simulink model "Adap_ob_CIDA_3_ODR_CFC"  (R2021b)
settings: Solver=ode5  StartTime=0.0  StopTime=90.0  FixedStep=0.02  RelTol=1e-3
settings Model: Creator=a1752760  LastModifiedBy=a1752760

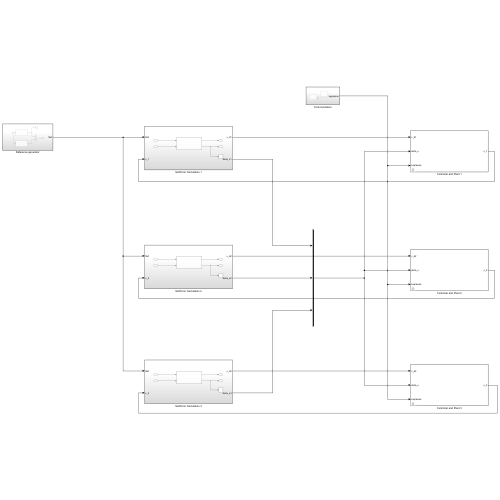
[thumbnail: Simulink's stored preview of the top-level diagram]
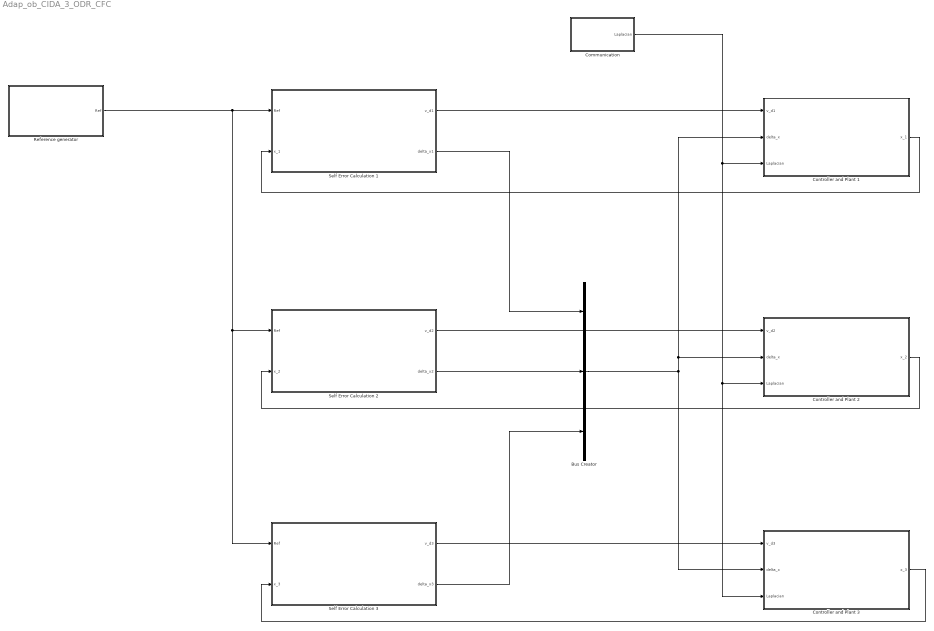
== system Adap_ob_CIDA_3_ODR_CFC ==
  Bus Creator : BusCreator  Inputs=3
  Communication : Subsystem
  Controller and Plant 1 : Subsystem  mask{InitialCondition=[-0.6;0.3;-pi/4], UpperLimit=0.2, LowerLimit=-0.2}
      mask prompts: InitialCondition "Simulink:blkprm_prompts:IntegratorInitCond"; UpperLimit "Simulink:blkprm_prompts:SaturateUpLim"; LowerLimit "Simulink:blkprm_prompts:SaturateLowLim"
      mask TypeOptions InitialCondition: x_int/InitialCondition
      mask TypeOptions UpperLimit: Saturation/UpperLimit
      mask TypeOptions LowerLimit: Saturation/LowerLimit
      mask DialogControl InitialCondition Prompt: Initial condition:
      mask DialogControl UpperLimit Prompt: Upper limit:
      mask DialogControl LowerLimit Prompt: Lower limit:
  Controller and Plant 2 : Subsystem  mask{InitialCondition=[0.1;1.4;pi/5], UpperLimit=0.2, LowerLimit=-0.2}
      mask prompts: InitialCondition "Simulink:blkprm_prompts:IntegratorInitCond"; UpperLimit "Simulink:blkprm_prompts:SaturateUpLim"; LowerLimit "Simulink:blkprm_prompts:SaturateLowLim"
      mask TypeOptions InitialCondition: x_int/InitialCondition
      mask TypeOptions UpperLimit: Saturation/UpperLimit
      mask TypeOptions LowerLimit: Saturation/LowerLimit
      mask DialogControl InitialCondition Prompt: Initial condition:
      mask DialogControl UpperLimit Prompt: Upper limit:
      mask DialogControl LowerLimit Prompt: Lower limit:
  Controller and Plant 3 : Subsystem  mask{InitialCondition=[1.1;0;pi/10], UpperLimit=0.2, LowerLimit=-0.2}
      mask prompts: InitialCondition "Simulink:blkprm_prompts:IntegratorInitCond"; UpperLimit "Simulink:blkprm_prompts:SaturateUpLim"; LowerLimit "Simulink:blkprm_prompts:SaturateLowLim"
      mask TypeOptions InitialCondition: x_int/InitialCondition
      mask TypeOptions UpperLimit: Saturation/UpperLimit
      mask TypeOptions LowerLimit: Saturation/LowerLimit
      mask DialogControl InitialCondition Prompt: Initial condition:
      mask DialogControl UpperLimit Prompt: Upper limit:
      mask DialogControl LowerLimit Prompt: Lower limit:
  Reference generator : Subsystem
  Self Error Calculation 1 : Subsystem
  Self Error Calculation 2 : Subsystem
  Self Error Calculation 3 : Subsystem
  wires:
  Communication/1(Laplacian) -> Controller and Plant 3/3(Laplacian), Controller and Plant 2/3(Laplacian), Controller and Plant 1/3(Laplacian)
  Self Error Calculation 1/2(delta_x1) -> Bus Creator/1
  Bus Creator/1 -> Controller and Plant 3/2(delta_x), Controller and Plant 2/2(delta_x), Controller and Plant 1/2(delta_x)
  Self Error Calculation 2/1(v_d2) -> Controller and Plant 2/1(v_d2)
  Self Error Calculation 2/2(delta_x2) -> Bus Creator/2
  Self Error Calculation 3/2(delta_x3) -> Bus Creator/3
  Self Error Calculation 3/1(v_d3) -> Controller and Plant 3/1(v_d3)
  Controller and Plant 2/1(x_2) -> Self Error Calculation 2/2(x_2)
  Controller and Plant 3/1(x_3) -> Self Error Calculation 3/2(x_3)
  Reference generator/1(Ref) -> Self Error Calculation 3/1(Ref), Self Error Calculation 2/1(Ref), Self Error Calculation 1/1(Ref)
  Controller and Plant 1/1(x_1) -> Self Error Calculation 1/2(x_1)
  Self Error Calculation 1/1(v_d1) -> Controller and Plant 1/1(v_d1)

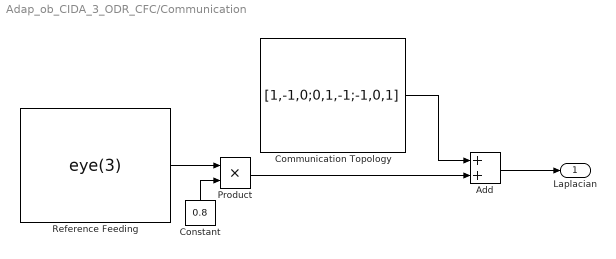
== system Adap_ob_CIDA_3_ODR_CFC/Communication ==
  Add : Sum
  Communication Topology : Constant  Value=[1,-1,0;0,1,-1;-1,0,1]  VectorParams1D=off
  Constant : Constant  Value=0.8  VectorParams1D=off
  Product : Product
  Reference Feeding : Constant  Value=eye(3)  VectorParams1D=off
  Laplacian : Outport  VectorParamsAs1DForOutWhenUnconnected=off
  wires:
  Constant/1 -> Product/2
  Reference Feeding/1 -> Product/1
  Communication Topology/1 -> Add/1
  Product/1 -> Add/2
  Add/1 -> Laplacian/1

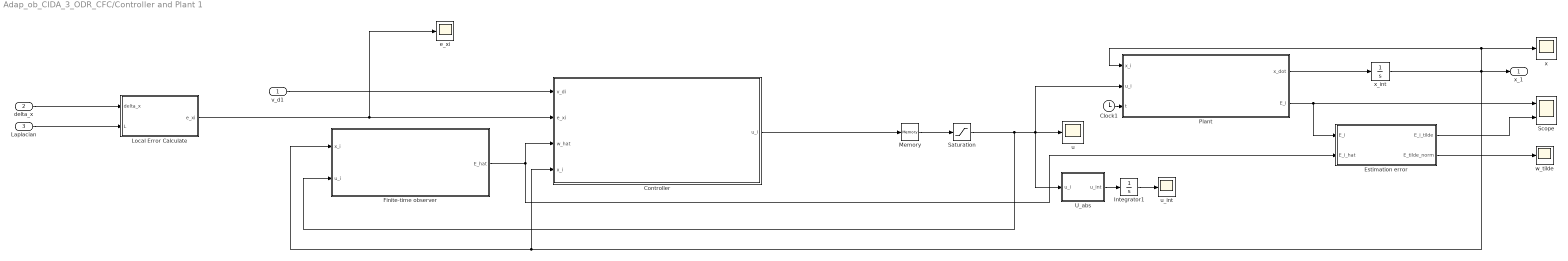
== system Adap_ob_CIDA_3_ODR_CFC/Controller and Plant 1 ==
  v_d1 : Inport
  delta_x : Inport  Port=2
  Laplacian : Inport  Port=3
  Clock1 : Clock
  Controller : Subsystem
  Estimation error : MATLAB Function  TreatAsAtomicUnit=on
  Finite-time observer : Subsystem  mask{InitialCondition=[-0.6;0.3;-pi/4]}
      mask prompts: InitialCondition "Simulink:blkprm_prompts:IntegratorInitCond"
      mask TypeOptions InitialCondition: Integrator/InitialCondition
      mask DialogControl InitialCondition Prompt: Initial condition:
  Integrator1 : Integrator
  Local Error Calculate : MATLAB Function  TreatAsAtomicUnit=on
  Memory : Memory  InitialCondition=[0;0;0]
  Plant : MATLAB Function  TreatAsAtomicUnit=on
  Saturation : Saturate  UpperLimit=UpperLimit  LowerLimit=LowerLimit
  Scope : Scope  NumInputPorts=2
  U_abs : MATLAB Function  TreatAsAtomicUnit=on
  e_xi : Scope
  u : Scope
  u_int : Scope
  w_tilde : Scope
  x : Scope
  x_int : Integrator  InitialCondition=InitialCondition
  x_1 : Outport
  wires:
  Plant/2(E_i) -> Scope/1, Estimation error/1(E_i)
  Finite-time observer/1(E_hat) -> Estimation error/2(E_i_hat), Controller/3(w_hat)
  Clock1/1 -> Plant/3(t)
  Plant/1(x_dot) -> x_int/1
  Memory/1 -> Saturation/1
  x_int/1 -> x_1/1, Plant/1(x_i), x/1, Finite-time observer/1(x_i), Controller/4(x_i)
  v_d1/1 -> Controller/1(v_di)
  Controller/1(u_i) -> Memory/1
  Local Error Calculate/1(e_xi) -> Controller/2(e_xi), e_xi/1
  delta_x/1 -> Local Error Calculate/1(delta_x)
  Laplacian/1 -> Local Error Calculate/2(L)
  Saturation/1 -> Finite-time observer/2(u_i), U_abs/1(u_i), Plant/2(u_i), u/1
  Integrator1/1 -> u_int/1
  U_abs/1(u_int) -> Integrator1/1
  Estimation error/2(E_tilde_norm) -> w_tilde/1
  Estimation error/1(E_i_tilde) -> Scope/2

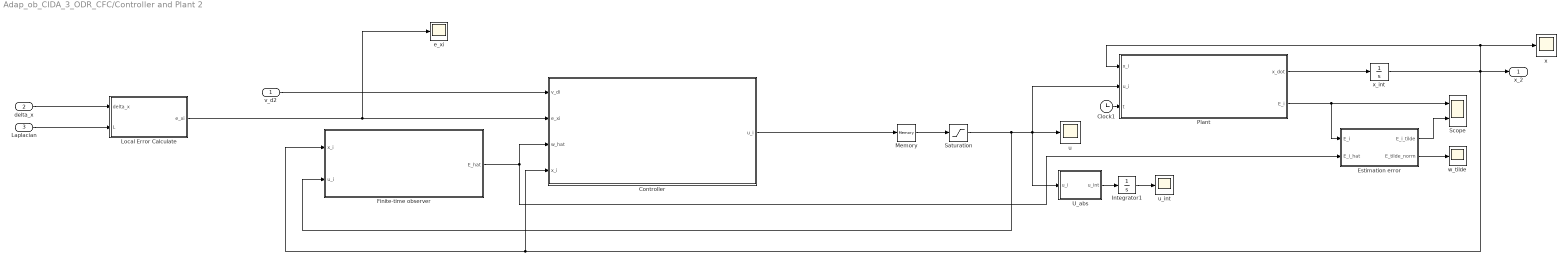
== system Adap_ob_CIDA_3_ODR_CFC/Controller and Plant 2 ==
  v_d2 : Inport
  delta_x : Inport  Port=2
  Laplacian : Inport  Port=3
  Clock1 : Clock
  Controller : Subsystem
  Estimation error : MATLAB Function  TreatAsAtomicUnit=on
  Finite-time observer : Subsystem  mask{InitialCondition=[0.1;1.4;pi/5]}
      mask prompts: InitialCondition "Simulink:blkprm_prompts:IntegratorInitCond"
      mask TypeOptions InitialCondition: Integrator/InitialCondition
      mask DialogControl InitialCondition Prompt: Initial condition:
  Integrator1 : Integrator
  Local Error Calculate : MATLAB Function  TreatAsAtomicUnit=on
  Memory : Memory  InitialCondition=[0;0;0]
  Plant : MATLAB Function  TreatAsAtomicUnit=on
  Saturation : Saturate  UpperLimit=UpperLimit  LowerLimit=LowerLimit
  Scope : Scope  NumInputPorts=2
  U_abs : MATLAB Function  TreatAsAtomicUnit=on
  e_xi : Scope
  u : Scope
  u_int : Scope
  w_tilde : Scope
  x : Scope
  x_int : Integrator  InitialCondition=InitialCondition
  x_2 : Outport
  wires:
  Plant/2(E_i) -> Estimation error/1(E_i), Scope/1
  Finite-time observer/1(E_hat) -> Controller/3(w_hat), Estimation error/2(E_i_hat)
  Clock1/1 -> Plant/3(t)
  Plant/1(x_dot) -> x_int/1
  Memory/1 -> Saturation/1
  x_int/1 -> x_2/1, Plant/1(x_i), x/1, Controller/4(x_i), Finite-time observer/1(x_i)
  v_d2/1 -> Controller/1(v_di)
  Controller/1(u_i) -> Memory/1
  Local Error Calculate/1(e_xi) -> Controller/2(e_xi), e_xi/1
  delta_x/1 -> Local Error Calculate/1(delta_x)
  Laplacian/1 -> Local Error Calculate/2(L)
  Integrator1/1 -> u_int/1
  Saturation/1 -> Finite-time observer/2(u_i), U_abs/1(u_i), Plant/2(u_i), u/1
  U_abs/1(u_int) -> Integrator1/1
  Estimation error/2(E_tilde_norm) -> w_tilde/1
  Estimation error/1(E_i_tilde) -> Scope/2

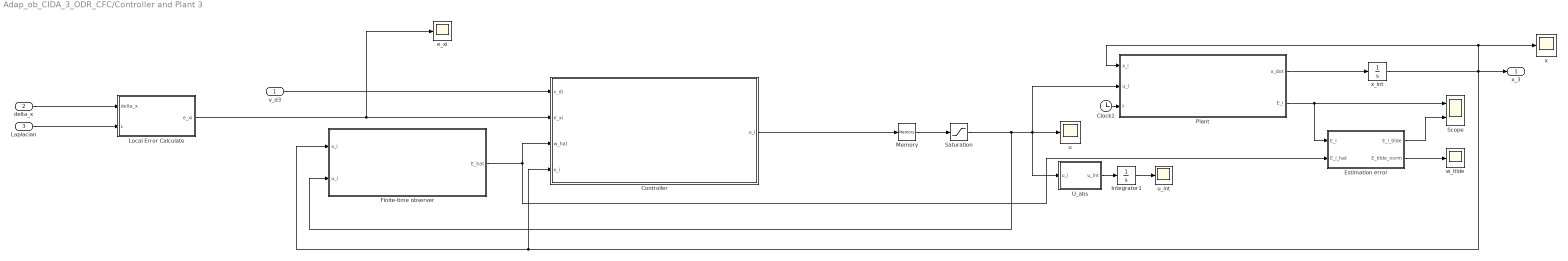
== system Adap_ob_CIDA_3_ODR_CFC/Controller and Plant 3 ==
  v_d3 : Inport
  delta_x : Inport  Port=2
  Laplacian : Inport  Port=3
  Clock1 : Clock
  Controller : Subsystem
  Estimation error : MATLAB Function  TreatAsAtomicUnit=on
  Finite-time observer : Subsystem  mask{InitialCondition=[1.1;0;pi/10]}
      mask prompts: InitialCondition "Simulink:blkprm_prompts:IntegratorInitCond"
      mask TypeOptions InitialCondition: Integrator/InitialCondition
      mask DialogControl InitialCondition Prompt: Initial condition:
  Integrator1 : Integrator
  Local Error Calculate : MATLAB Function  TreatAsAtomicUnit=on
  Memory : Memory  InitialCondition=[0;0;0]
  Plant : MATLAB Function  TreatAsAtomicUnit=on
  Saturation : Saturate  UpperLimit=UpperLimit  LowerLimit=LowerLimit
  Scope : Scope  NumInputPorts=2
  U_abs : MATLAB Function  TreatAsAtomicUnit=on
  e_xi : Scope
  u : Scope
  u_int : Scope
  w_tilde : Scope
  x : Scope
  x_int : Integrator  InitialCondition=InitialCondition
  x_3 : Outport
  wires:
  Plant/2(E_i) -> Scope/1, Estimation error/1(E_i)
  Finite-time observer/1(E_hat) -> Controller/3(w_hat), Estimation error/2(E_i_hat)
  Clock1/1 -> Plant/3(t)
  Plant/1(x_dot) -> x_int/1
  Memory/1 -> Saturation/1
  x_int/1 -> x_3/1, Plant/1(x_i), x/1, Controller/4(x_i), Finite-time observer/1(x_i)
  v_d3/1 -> Controller/1(v_di)
  Controller/1(u_i) -> Memory/1
  Local Error Calculate/1(e_xi) -> Controller/2(e_xi), e_xi/1
  delta_x/1 -> Local Error Calculate/1(delta_x)
  Laplacian/1 -> Local Error Calculate/2(L)
  Integrator1/1 -> u_int/1
  Saturation/1 -> Finite-time observer/2(u_i), U_abs/1(u_i), Plant/2(u_i), u/1
  U_abs/1(u_int) -> Integrator1/1
  Estimation error/2(E_tilde_norm) -> w_tilde/1
  Estimation error/1(E_i_tilde) -> Scope/2

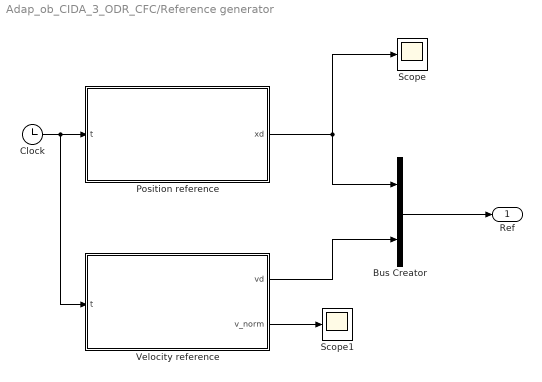
== system Adap_ob_CIDA_3_ODR_CFC/Reference generator ==
  Bus Creator : BusCreator  Inputs=2
  Clock : Clock
  Position reference : MATLAB Function  TreatAsAtomicUnit=on
  Scope : Scope
  Scope1 : Scope
  Velocity reference : MATLAB Function  TreatAsAtomicUnit=on
  Ref : Outport
  wires:
  Clock/1 -> Velocity reference/1(t), Position reference/1(t)
  Position reference/1(xd) -> Scope/1, Bus Creator/1
  Velocity reference/1(vd) -> Bus Creator/2
  Bus Creator/1 -> Ref/1
  Velocity reference/2(v_norm) -> Scope1/1

== system Adap_ob_CIDA_3_ODR_CFC/Self Error Calculation 1 ==
  Ref : Inport
  x_1 : Inport  Port=2
  Scope : Scope
  error_calculation : MATLAB Function  TreatAsAtomicUnit=on
  v_d1 : Outport
  delta_x1 : Outport  Port=2
  wires:
  Ref/1 -> error_calculation/1(ref)
  x_1/1 -> error_calculation/2(x_i)
  error_calculation/1(v_di) -> v_d1/1
  error_calculation/2(delta_x1) -> Scope/1, delta_x1/1

== system Adap_ob_CIDA_3_ODR_CFC/Self Error Calculation 2 ==
  Ref : Inport
  x_2 : Inport  Port=2
  Scope : Scope
  error_calculation : MATLAB Function  TreatAsAtomicUnit=on
  v_d2 : Outport
  delta_x2 : Outport  Port=2
  wires:
  Ref/1 -> error_calculation/1(ref)
  x_2/1 -> error_calculation/2(x_i)
  error_calculation/1(v_di) -> v_d2/1
  error_calculation/2(delta_x2) -> Scope/1, delta_x2/1

== system Adap_ob_CIDA_3_ODR_CFC/Self Error Calculation 3 ==
  Ref : Inport
  x_3 : Inport  Port=2
  Scope : Scope
  error_calculation : MATLAB Function  TreatAsAtomicUnit=on
  v_d3 : Outport
  delta_x3 : Outport  Port=2
  wires:
  Ref/1 -> error_calculation/1(ref)
  x_3/1 -> error_calculation/2(x_i)
  error_calculation/1(v_di) -> v_d3/1
  error_calculation/2(delta_x3) -> Scope/1, delta_x3/1

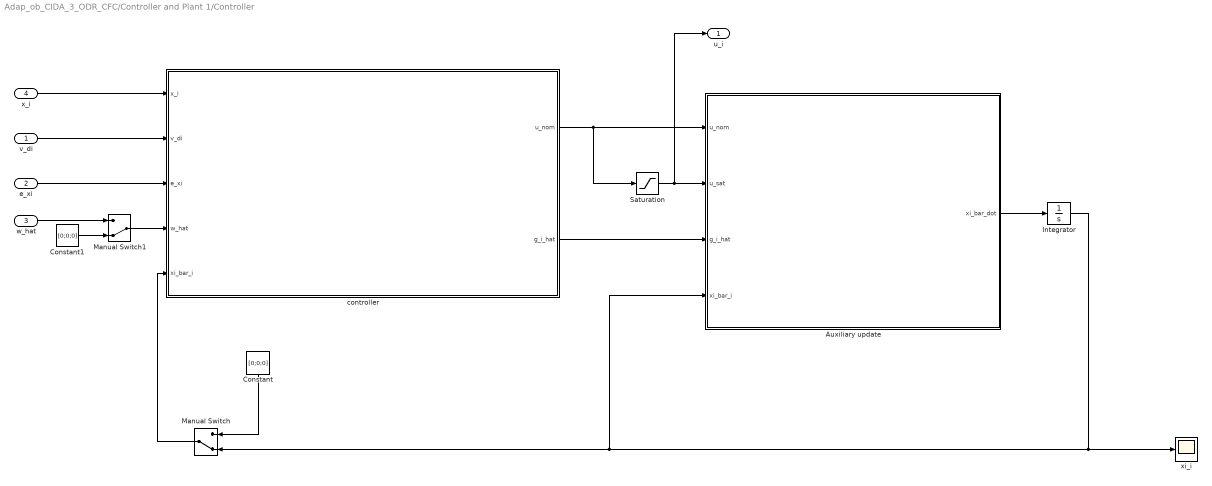
== system Adap_ob_CIDA_3_ODR_CFC/Controller and Plant 1/Controller ==
  v_di : Inport
  e_xi : Inport  Port=2
  w_hat : Inport  Port=3
  x_i : Inport  Port=4
  Auxiliary update : MATLAB Function  TreatAsAtomicUnit=on
  Constant : Constant  Value=[0;0;0]
  Constant1 : Constant  Value=[0;0;0]  VectorParams1D=off
  Integrator : Integrator  InitialCondition=[0;0;0]
  Manual Switch : ManualSwitch  CurrentSetting=0
  Manual Switch1 : ManualSwitch  CurrentSetting=0
  Saturation : Saturate  UpperLimit=0.2  LowerLimit=-0.2
  controller : MATLAB Function  TreatAsAtomicUnit=on
  xi_i : Scope
  u_i : Outport
  wires:
  x_i/1 -> controller/1(x_i)
  v_di/1 -> controller/2(v_di)
  e_xi/1 -> controller/3(e_xi)
  controller/1(u_nom) -> Saturation/1, Auxiliary update/1(u_nom)
  Saturation/1 -> u_i/1, Auxiliary update/2(u_sat)
  controller/2(g_i_hat) -> Auxiliary update/3(g_i_hat)
  Auxiliary update/1(xi_bar_dot) -> Integrator/1
  Constant/1 -> Manual Switch/1
  Manual Switch/1 -> controller/5(xi_bar_i)
  Integrator/1 -> xi_i/1, Auxiliary update/4(xi_bar_i), Manual Switch/2
  Constant1/1 -> Manual Switch1/2
  Manual Switch1/1 -> controller/4(w_hat)
  w_hat/1 -> Manual Switch1/1

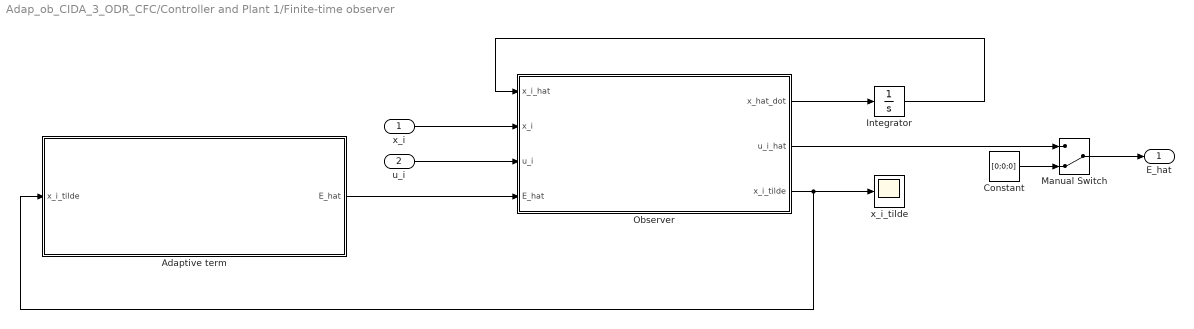
== system Adap_ob_CIDA_3_ODR_CFC/Controller and Plant 1/Finite-time observer ==
  x_i : Inport
  u_i : Inport  Port=2
  Adaptive term : Subsystem
  Constant : Constant  Value=[0;0;0]  VectorParams1D=off
  Integrator : Integrator  InitialCondition=InitialCondition
  Manual Switch : ManualSwitch  CurrentSetting=0
  Observer : MATLAB Function  TreatAsAtomicUnit=on
  x_i_tilde : Scope
  E_hat : Outport
  wires:
  x_i/1 -> Observer/2(x_i)
  u_i/1 -> Observer/3(u_i)
  Adaptive term/1(E_hat) -> Observer/4(E_hat)
  Observer/1(x_hat_dot) -> Integrator/1
  Integrator/1 -> Observer/1(x_i_hat)
  Observer/3(x_i_tilde) -> x_i_tilde/1, Adaptive term/1(x_i_tilde)
  Observer/2(u_i_hat) -> Manual Switch/1
  Manual Switch/1 -> E_hat/1
  Constant/1 -> Manual Switch/2

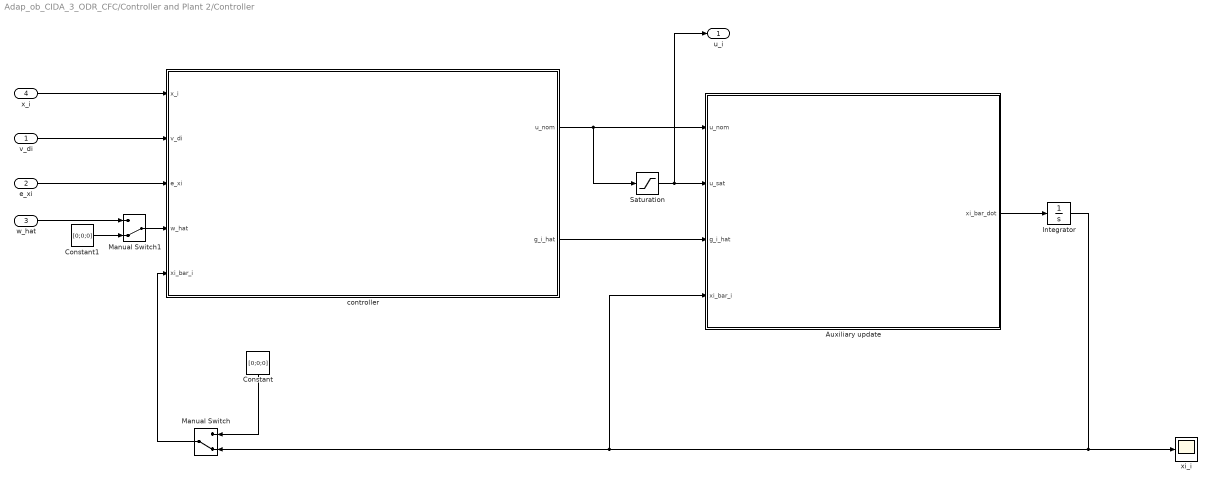
== system Adap_ob_CIDA_3_ODR_CFC/Controller and Plant 2/Controller ==
  v_di : Inport
  e_xi : Inport  Port=2
  w_hat : Inport  Port=3
  x_i : Inport  Port=4
  Auxiliary update : MATLAB Function  TreatAsAtomicUnit=on
  Constant : Constant  Value=[0;0;0]
  Constant1 : Constant  Value=[0;0;0]  VectorParams1D=off
  Integrator : Integrator  InitialCondition=[0;0;0]
  Manual Switch : ManualSwitch  CurrentSetting=0
  Manual Switch1 : ManualSwitch  CurrentSetting=0
  Saturation : Saturate  UpperLimit=0.2  LowerLimit=-0.2
  controller : MATLAB Function  TreatAsAtomicUnit=on
  xi_i : Scope
  u_i : Outport
  wires:
  x_i/1 -> controller/1(x_i)
  v_di/1 -> controller/2(v_di)
  e_xi/1 -> controller/3(e_xi)
  controller/1(u_nom) -> Saturation/1, Auxiliary update/1(u_nom)
  Saturation/1 -> u_i/1, Auxiliary update/2(u_sat)
  controller/2(g_i_hat) -> Auxiliary update/3(g_i_hat)
  Auxiliary update/1(xi_bar_dot) -> Integrator/1
  Constant/1 -> Manual Switch/1
  Manual Switch/1 -> controller/5(xi_bar_i)
  Integrator/1 -> xi_i/1, Auxiliary update/4(xi_bar_i), Manual Switch/2
  Constant1/1 -> Manual Switch1/2
  Manual Switch1/1 -> controller/4(w_hat)
  w_hat/1 -> Manual Switch1/1

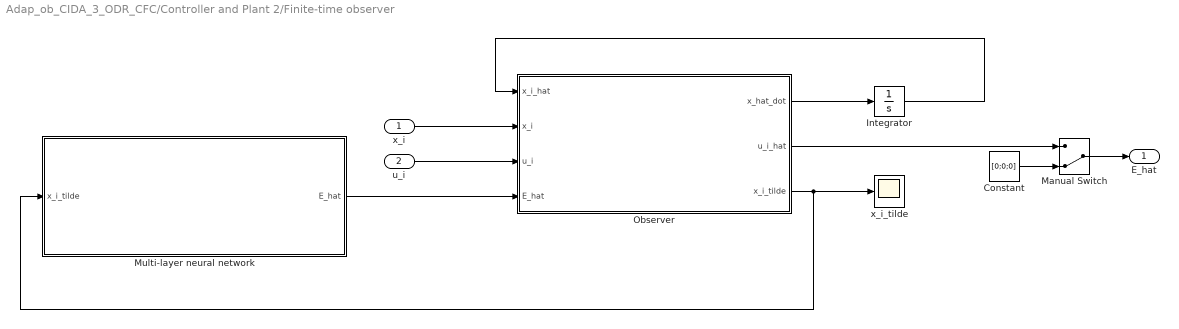
== system Adap_ob_CIDA_3_ODR_CFC/Controller and Plant 2/Finite-time observer ==
  x_i : Inport
  u_i : Inport  Port=2
  Constant : Constant  Value=[0;0;0]  VectorParams1D=off
  Integrator : Integrator  InitialCondition=InitialCondition
  Manual Switch : ManualSwitch  CurrentSetting=0
  Multi-layer neural network : Subsystem
  Observer : MATLAB Function  TreatAsAtomicUnit=on
  x_i_tilde : Scope
  E_hat : Outport
  wires:
  x_i/1 -> Observer/2(x_i)
  u_i/1 -> Observer/3(u_i)
  Multi-layer neural network/1(E_hat) -> Observer/4(E_hat)
  Observer/1(x_hat_dot) -> Integrator/1
  Integrator/1 -> Observer/1(x_i_hat)
  Observer/3(x_i_tilde) -> x_i_tilde/1, Multi-layer neural network/1(x_i_tilde)
  Observer/2(u_i_hat) -> Manual Switch/1
  Constant/1 -> Manual Switch/2
  Manual Switch/1 -> E_hat/1

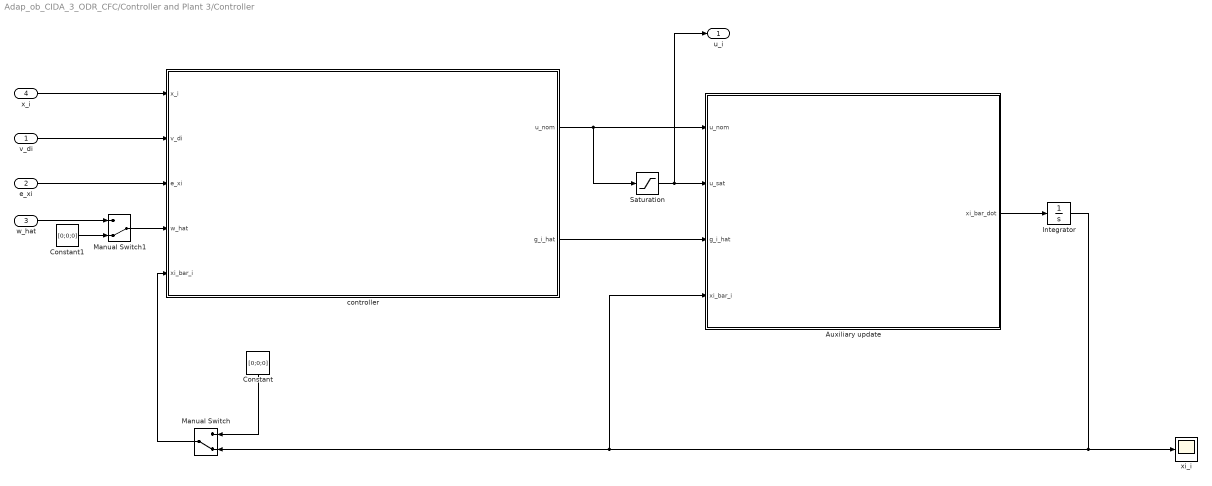
== system Adap_ob_CIDA_3_ODR_CFC/Controller and Plant 3/Controller ==
  v_di : Inport
  e_xi : Inport  Port=2
  w_hat : Inport  Port=3
  x_i : Inport  Port=4
  Auxiliary update : MATLAB Function  TreatAsAtomicUnit=on
  Constant : Constant  Value=[0;0;0]
  Constant1 : Constant  Value=[0;0;0]  VectorParams1D=off
  Integrator : Integrator  InitialCondition=[0;0;0]
  Manual Switch : ManualSwitch  CurrentSetting=0
  Manual Switch1 : ManualSwitch  CurrentSetting=0
  Saturation : Saturate  UpperLimit=0.2  LowerLimit=-0.2
  controller : MATLAB Function  TreatAsAtomicUnit=on
  xi_i : Scope
  u_i : Outport
  wires:
  x_i/1 -> controller/1(x_i)
  v_di/1 -> controller/2(v_di)
  e_xi/1 -> controller/3(e_xi)
  controller/1(u_nom) -> Saturation/1, Auxiliary update/1(u_nom)
  Saturation/1 -> u_i/1, Auxiliary update/2(u_sat)
  controller/2(g_i_hat) -> Auxiliary update/3(g_i_hat)
  Auxiliary update/1(xi_bar_dot) -> Integrator/1
  Constant/1 -> Manual Switch/1
  Manual Switch/1 -> controller/5(xi_bar_i)
  Integrator/1 -> xi_i/1, Auxiliary update/4(xi_bar_i), Manual Switch/2
  Constant1/1 -> Manual Switch1/2
  w_hat/1 -> Manual Switch1/1
  Manual Switch1/1 -> controller/4(w_hat)

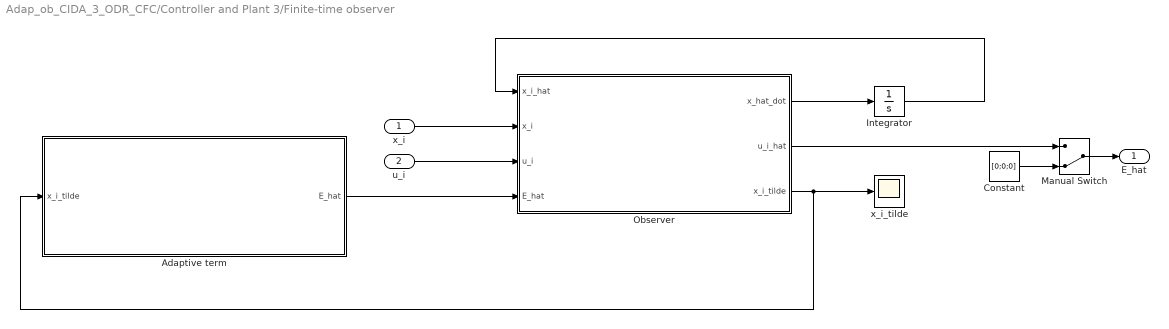
== system Adap_ob_CIDA_3_ODR_CFC/Controller and Plant 3/Finite-time observer ==
  x_i : Inport
  u_i : Inport  Port=2
  Adaptive term : Subsystem
  Constant : Constant  Value=[0;0;0]  VectorParams1D=off
  Integrator : Integrator  InitialCondition=InitialCondition
  Manual Switch : ManualSwitch  CurrentSetting=0
  Observer : MATLAB Function  TreatAsAtomicUnit=on
  x_i_tilde : Scope
  E_hat : Outport
  wires:
  x_i/1 -> Observer/2(x_i)
  u_i/1 -> Observer/3(u_i)
  Adaptive term/1(E_hat) -> Observer/4(E_hat)
  Observer/1(x_hat_dot) -> Integrator/1
  Integrator/1 -> Observer/1(x_i_hat)
  Observer/3(x_i_tilde) -> x_i_tilde/1, Adaptive term/1(x_i_tilde)
  Observer/2(u_i_hat) -> Manual Switch/1
  Constant/1 -> Manual Switch/2
  Manual Switch/1 -> E_hat/1

== system Adap_ob_CIDA_3_ODR_CFC/Controller and Plant 1/Finite-time observer/Adaptive term ==
  x_i_tilde : Inport
  E_dot : Integrator  InitialCondition=[0;0;0]
  E_hat_1 : Scope
  Update law : MATLAB Function  TreatAsAtomicUnit=on
  E_hat : Outport
  wires:
  E_dot/1 -> Update law/2(E_hat_prev), E_hat/1, E_hat_1/1
  x_i_tilde/1 -> Update law/1(x_tilde)
  Update law/1(dot_E_hat) -> E_dot/1

== system Adap_ob_CIDA_3_ODR_CFC/Controller and Plant 2/Finite-time observer/Multi-layer neural network ==
  x_i_tilde : Inport
  E_dot : Integrator  InitialCondition=[0;0;0]
  E_hat_1 : Scope
  Update law : MATLAB Function  TreatAsAtomicUnit=on
  E_hat : Outport
  wires:
  E_dot/1 -> Update law/2(E_hat_prev), E_hat/1, E_hat_1/1
  x_i_tilde/1 -> Update law/1(x_tilde)
  Update law/1(dot_E_hat) -> E_dot/1

== system Adap_ob_CIDA_3_ODR_CFC/Controller and Plant 3/Finite-time observer/Adaptive term ==
  x_i_tilde : Inport
  E_dot : Integrator  InitialCondition=[0;0;0]
  E_hat_1 : Scope
  Update law : MATLAB Function  TreatAsAtomicUnit=on
  E_hat : Outport
  wires:
  E_dot/1 -> Update law/2(E_hat_prev), E_hat/1, E_hat_1/1
  x_i_tilde/1 -> Update law/1(x_tilde)
  Update law/1(dot_E_hat) -> E_dot/1

== matlab function Adap_ob_CIDA_3_ODR_CFC/Controller and Plant 2/Finite-time observer/Multi-layer neural network/Update law ==
  data: x_tilde input; dot_E_hat output; E_hat_prev input
function dot_E_hat = adaptive_law(x_tilde, E_hat_prev)

eta_5 = diag([10,10,3]);
eta_6 = 1.1;
dot_E_hat = eta_5 * x_tilde - eta_6 * E_hat_prev;

end

== matlab function Adap_ob_CIDA_3_ODR_CFC/Controller and Plant 2/Finite-time observer/Observer ==
  data: x_i_hat input; x_i input; u_i input; x_hat_dot output; u_i_hat output; E_hat input; x_i_tilde output
function [x_hat_dot, u_i_hat, x_i_tilde] = observer(x_i_hat, x_i, u_i, E_hat)

%% observer itself
Radius=[0.134;0.128;0.126];
Radius_esti=[0.13,0.13,0.13];

serial_num = 2;
dimension = 3; 

k_1 = diag([2.2,2.2,0.4]);
k_2 = diag([0.8,0.8,0.4]);

p = 9/11;

R_hat=Radius_esti(serial_num);

theta = x_i(dimension);

g_i_hat = [-sin(theta) -sin(pi/3 - theta) sin(pi/3 + theta);
            cos(theta) -cos(pi/3 - theta) -cos(pi/3+ theta);
            1/R_hat 1/R_hat 1/R_hat];

x_i_tilde = x_i - x_i_hat;

u_i_hat = E_hat + k_1 * x_i_tilde + k_2 * diag(sign(x_i_tilde)) * abs(x_i_tilde).^p;

x_hat_dot = g_i_hat * u_i + u_i_hat;

end

== matlab function Adap_ob_CIDA_3_ODR_CFC/Controller and Plant 3/Controller/Auxiliary update ==
  data: u_nom input; xi_bar_dot output; u_sat input; g_i_hat input; xi_bar_i input
function xi_bar_dot = auxi_updata(u_nom, u_sat, g_i_hat, xi_bar_i)

eta_3 = diag([6,6,1]);

u_diff = u_nom - u_sat;

eta_4 = diag([0.5,0.5,0.2]);

% if norm(u_diff) == 0
%     eta_8 = diag([2,2,2]);
% else
%     eta_8 = diag([0.5,0.5,0.2]);
% end

xi_bar_dot = eta_3 * g_i_hat * u_diff - eta_4 * xi_bar_i;

end

== matlab function Adap_ob_CIDA_3_ODR_CFC/Controller and Plant 1/Local Error Calculate ==
  data: delta_x input; e_xi output; L input
function e_xi = local_error(delta_x, L)

%% Calculate the local formation tracking error from communication

dimension = 3;
serial_num = 1;

L_i = kron(L(serial_num, :) , eye(dimension));

e_xi = L_i * delta_x;

end

== matlab function Adap_ob_CIDA_3_ODR_CFC/Controller and Plant 2/Local Error Calculate ==
  data: delta_x input; e_xi output; L input
function e_xi = local_error(delta_x, L)

%% Calculate the local formation tracking error from communication

dimension = 3;
serial_num = 2;

L_i = kron(L(serial_num, :) , eye(dimension));

e_xi = L_i * delta_x;







end

== matlab function Adap_ob_CIDA_3_ODR_CFC/Controller and Plant 3/Finite-time observer/Adaptive term/Update law ==
  data: x_tilde input; dot_E_hat output; E_hat_prev input
function dot_E_hat = adaptive_law(x_tilde, E_hat_prev)

eta_5 = diag([10,10,3]);
eta_6 = 1.1;
dot_E_hat = eta_5 * x_tilde - eta_6 * E_hat_prev;

end

== matlab function Adap_ob_CIDA_3_ODR_CFC/Controller and Plant 3/Finite-time observer/Observer ==
  data: x_i_hat input; x_i input; u_i input; x_hat_dot output; u_i_hat output; E_hat input; x_i_tilde output
function [x_hat_dot, u_i_hat, x_i_tilde] = observer(x_i_hat, x_i, u_i, E_hat)

%% observer itself
Radius=[0.134;0.128;0.126];
Radius_esti=[0.13,0.13,0.13];

serial_num = 3;
dimension = 3; 

k_1 = diag([2.2,2.2,0.4]);
k_2 = diag([0.8,0.8,0.4]);

p = 9/11;

R_hat=Radius_esti(serial_num);

theta = x_i(dimension);

g_i_hat = [-sin(theta) -sin(pi/3 - theta) sin(pi/3 + theta);
            cos(theta) -cos(pi/3 - theta) -cos(pi/3+ theta);
            1/R_hat 1/R_hat 1/R_hat];

x_i_tilde = x_i - x_i_hat;

u_i_hat = E_hat + k_1 * x_i_tilde + k_2 * diag(sign(x_i_tilde)) * abs(x_i_tilde).^p;

x_hat_dot = g_i_hat * u_i + u_i_hat;


end

== matlab function Adap_ob_CIDA_3_ODR_CFC/Controller and Plant 3/Controller/controller ==
  data: x_i input; v_di input; u_nom output; e_xi input; w_hat input; xi_bar_i input; g_i_hat output
function [u_nom, g_i_hat] = controller(x_i, v_di, e_xi, w_hat, xi_bar_i)

%% Reverse of the control gain matrix
Radius_esti=[0.13,0.13,0.13];

serial_num = 3;
dimension = 3; 

R_hat=Radius_esti(serial_num);

theta = x_i(dimension);

g_i_hat = [-sin(theta) -sin(pi/3 - theta) sin(pi/3 + theta);
        cos(theta) -cos(pi/3 - theta) -cos(pi/3+ theta);
        1/R_hat 1/R_hat 1/R_hat];

g_inverse = g_i_hat^(-1); 

%% Nominal control input
k_e = diag([1.6,1.6,1.6]);
k_xi = diag([8,8,2]);

u_nom = g_inverse * (- k_e * e_xi - k_xi * xi_bar_i - w_hat + v_di);

end

== matlab function Adap_ob_CIDA_3_ODR_CFC/Controller and Plant 2/Plant ==
  data: x_dot output; E_i output; x_i input; u_i input; t input
function [x_dot, E_i ] = model(x_i, u_i, t)

%% First-order plants for robots

Radius=[0.13,0.13,0.13];
Radius_esti=[0.13,0.13,0.13];

serial_num = 2;
dimension = 3; 

R = Radius(serial_num);
R_hat = Radius_esti(serial_num);

x = x_i(1);
y = x_i(2);
theta = x_i(3);

w_i =  [0.08 * cos(0.5* t+ serial_num * pi/2); 0.09 * sin(0.2*t + serial_num * pi/3); 0.08*sin(0.1*t + serial_num * pi/4)];
%d =  0.4* cos(0.5* t+ pi/2);


g_i = [-sin(theta) -sin(pi/3 - theta) sin(pi/3 + theta);
        cos(theta) -cos(pi/3 - theta) -cos(pi/3+ theta);
        1/R 1/R 1/R];
    
g_i_hat = [-sin(theta) -sin(pi/3 - theta) sin(pi/3 + theta);
        cos(theta) -cos(pi/3 - theta) -cos(pi/3+ theta);
        1/R_hat 1/R_hat 1/R_hat];
    
x_dot = g_i * u_i + w_i;


E_i = w_i + (g_i - g_i_hat) * u_i;




end

== matlab function Adap_ob_CIDA_3_ODR_CFC/Self Error Calculation 2/error_calculation ==
  data: v_di output; ref input; delta_x2 output; x_i input
function [v_di, delta_x2] = error_cal(ref, x_i)

%% Basic parameters

dimension = 3;
num_agent = 3;
serial_num = 2;

x_d = ref(1+dimension*0:dimension*num_agent);
v_d = ref(1+dimension*num_agent:2*dimension*num_agent);

x_di = x_d( (serial_num - 1)*dimension+1 : serial_num*dimension );
v_di = v_d( (serial_num - 1)*dimension+1 : serial_num*dimension );

delta_x2 = x_i - x_di;

end

== matlab function Adap_ob_CIDA_3_ODR_CFC/Controller and Plant 3/Local Error Calculate ==
  data: delta_x input; e_xi output; L input
function e_xi = local_error(delta_x, L)

%% Calculate the local formation tracking error from communication

dimension = 3;
serial_num = 3;

L_i = kron(L(serial_num, :) , eye(dimension));

e_xi = L_i * delta_x;







end

== matlab function Adap_ob_CIDA_3_ODR_CFC/Controller and Plant 1/Controller/Auxiliary update ==
  data: u_nom input; xi_bar_dot output; u_sat input; g_i_hat input; xi_bar_i input
function xi_bar_dot = auxi_updata(u_nom, u_sat, g_i_hat, xi_bar_i)

eta_3 = diag([6,6,1]);

u_diff = u_nom - u_sat;

eta_4 = diag([0.5,0.5,0.2]);

% if norm(u_diff) == 0
%     eta_8 = diag([2,2,2]);
% else
%     eta_8 = diag([0.5,0.5,0.2]);
% end

xi_bar_dot = eta_3 * g_i_hat * u_diff - eta_4 * xi_bar_i;

end

== matlab function Adap_ob_CIDA_3_ODR_CFC/Self Error Calculation 3/error_calculation ==
  data: v_di output; ref input; delta_x3 output; x_i input
function [v_di, delta_x3] = error_cal(ref, x_i)

%% Basic parameters

dimension = 3;
num_agent = 3;
serial_num = 3;

x_d = ref(1+dimension*0:dimension*num_agent);
v_d = ref(1+dimension*num_agent:2*dimension*num_agent);

x_di = x_d( (serial_num - 1)*dimension+1 : serial_num*dimension );
v_di = v_d( (serial_num - 1)*dimension+1 : serial_num*dimension );

delta_x3 = x_i - x_di;

end

== matlab function Adap_ob_CIDA_3_ODR_CFC/Controller and Plant 3/Plant ==
  data: x_dot output; E_i output; x_i input; u_i input; t input
function [x_dot, E_i ] = model( x_i, u_i, t)

%% First-order plants for robots
Radius=[0.13,0.13,0.13];
Radius_esti=[0.13,0.13,0.13];

serial_num = 3;
dimension = 3; 

R = Radius(serial_num);
R_hat = Radius_esti(serial_num);

x = x_i(1);
y = x_i(2);
theta = x_i(3);

w_i =  [0.08 * cos(0.5* t+ serial_num * pi/2); 0.09 * sin(0.2*t + serial_num * pi/3); 0.08*sin(0.1*t + serial_num * pi/4)];
%d =  0.4* cos(0.5* t+ pi/2);


g_i = [-sin(theta) -sin(pi/3 - theta) sin(pi/3 + theta);
        cos(theta) -cos(pi/3 - theta) -cos(pi/3+ theta);
        1/R 1/R 1/R];
    
g_i_hat = [-sin(theta) -sin(pi/3 - theta) sin(pi/3 + theta);
            cos(theta) -cos(pi/3 - theta) -cos(pi/3+ theta);
            1/R_hat 1/R_hat 1/R_hat];
    
x_dot = g_i * u_i + w_i;


E_i = w_i + (g_i - g_i_hat) * u_i;




end

== matlab function Adap_ob_CIDA_3_ODR_CFC/Controller and Plant 1/Finite-time observer/Observer ==
  data: x_i_hat input; x_i input; u_i input; x_hat_dot output; u_i_hat output; E_hat input; x_i_tilde output
function [x_hat_dot, u_i_hat, x_i_tilde] = observer(x_i_hat, x_i, u_i, E_hat)

%% observer itself
Radius=[0.134;0.128;0.126];
Radius_esti=[0.13,0.13,0.13];

serial_num = 1;
dimension = 3; 

k_1 = diag([2.2,2.2,0.4]);
k_2 = diag([0.8,0.8,0.4]);

p = 9/11;

R_hat=Radius_esti(serial_num);

theta = x_i(dimension);

g_i_hat = [-sin(theta) -sin(pi/3 - theta) sin(pi/3 + theta);
            cos(theta) -cos(pi/3 - theta) -cos(pi/3+ theta);
            1/R_hat 1/R_hat 1/R_hat];

x_i_tilde = x_i - x_i_hat;

u_i_hat = E_hat + k_1 * x_i_tilde + k_2 * diag(sign(x_i_tilde)) * abs(x_i_tilde).^p;

x_hat_dot = g_i_hat * u_i + u_i_hat;

end

== matlab function Adap_ob_CIDA_3_ODR_CFC/Controller and Plant 1/Controller/controller ==
  data: x_i input; v_di input; u_nom output; e_xi input; w_hat input; xi_bar_i input; g_i_hat output
function [u_nom, g_i_hat] = controller(x_i, v_di, e_xi, w_hat, xi_bar_i)

%% Reverse of the control gain matrix
Radius_esti=[0.13,0.13,0.13];

serial_num = 1;
dimension = 3; 

R_hat=Radius_esti(serial_num);

theta = x_i(dimension);

g_i_hat = [-sin(theta) -sin(pi/3 - theta) sin(pi/3 + theta);
        cos(theta) -cos(pi/3 - theta) -cos(pi/3+ theta);
        1/R_hat 1/R_hat 1/R_hat];

g_inverse = g_i_hat^(-1); 

%% Nominal control input
k_e = diag([1.6,1.6,1.6]);
k_xi = diag([8,8,2]);

u_nom = g_inverse * (- k_e * e_xi - k_xi * xi_bar_i - w_hat + v_di);

end

== matlab function Adap_ob_CIDA_3_ODR_CFC/Controller and Plant 3/U_abs ==
  data: u_i input; u_int output
function  u_int = fcn(u_i)

u_ab = abs(u_i);

u_int = u_ab(1) + u_ab(2) + u_ab(3);


end

== matlab function Adap_ob_CIDA_3_ODR_CFC/Controller and Plant 2/U_abs ==
  data: u_i input; u_int output
function  u_int = fcn(u_i)

u_ab = abs(u_i);

u_int = u_ab(1) + u_ab(2) + u_ab(3);


end

== matlab function Adap_ob_CIDA_3_ODR_CFC/Controller and Plant 1/U_abs ==
  data: u_i input; u_int output
function  u_int = fcn(u_i)

u_ab = abs(u_i);

u_int = u_ab(1) + u_ab(2) + u_ab(3);


end

== matlab function Adap_ob_CIDA_3_ODR_CFC/Reference generator/Position reference ==
  data: t input; xd output
function xd = x_d(t)

% bias_x=0.2*t;
% bias_y=sin(0.3*t);

bias_x= 0.2 * sin(pi/15 * t);
bias_y= - t/30 + 0.8;

radius=0.8;
w=pi/20;

phase=0;

x1=[radius*cos(w*t+2*pi/3*1+phase)+bias_x ; radius*sin(w*t+2*pi/3*1+phase)+bias_y ; 0];
x2=[radius*cos(w*t+2*pi/3*2+phase)+bias_x ; radius*sin(w*t+2*pi/3*2+phase)+bias_y ; 0];
x3=[radius*cos(w*t+2*pi/3*3+phase)+bias_x ; radius*sin(w*t+2*pi/3*3+phase)+bias_y ; 0];

xd=[x1;x2;x3];

end

== matlab function Adap_ob_CIDA_3_ODR_CFC/Reference generator/Velocity reference ==
  data: t input; vd output; v_norm output
function [vd, v_norm] = v_d(t)

bias_x_v = 0.2 * pi /15 * cos(pi/15 * t);
bias_y_v = - 1/30;

radius=0.8;
w=pi/20;

phase = 0;

v1=[- radius * w * sin(w*t+2*pi/3*1+phase)+bias_x_v; radius * w * cos(w*t+2*pi/3*1+phase) + bias_y_v; 0];
v2=[- radius * w * sin(w*t+2*pi/3*2+phase)+bias_x_v; radius * w * cos(w*t+2*pi/3*2+phase) + bias_y_v; 0];
v3=[- radius * w * sin(w*t+2*pi/3*3+phase)+bias_x_v; radius * w * cos(w*t+2*pi/3*3+phase) + bias_y_v; 0];

vd=[v1;v2;v3];

v_norm = norm(v3);

end

== matlab function Adap_ob_CIDA_3_ODR_CFC/Controller and Plant 1/Plant ==
  data: x_dot output; E_i output; x_i input; u_i input; t input
function [x_dot, E_i ] = model(x_i, u_i, t)

%% First-order plants for robots
Radius=[0.13,0.13,0.13];
Radius_esti=[0.13,0.13,0.13];

serial_num = 1;

R = Radius(serial_num);
R_hat = Radius_esti(serial_num);

x = x_i(1);
y = x_i(2);
theta = x_i(3);

w_i =  [0.08 * cos(0.5* t+ serial_num * pi/2); 0.09 * sin(0.2*t + serial_num * pi/3); 0.08*sin(0.1*t + serial_num * pi/4)];
%d =  0.4* cos(0.5* t+ pi/2);


g_i = [-sin(theta) -sin(pi/3 - theta) sin(pi/3 + theta);
        cos(theta) -cos(pi/3 - theta) -cos(pi/3+ theta);
        1/R 1/R 1/R];
    
g_i_hat = [-sin(theta) -sin(pi/3 - theta) sin(pi/3 + theta);
        cos(theta) -cos(pi/3 - theta) -cos(pi/3+ theta);
        1/R_hat 1/R_hat 1/R_hat];
    
x_dot = g_i * u_i + w_i;


E_i = w_i + (g_i - g_i_hat) * u_i;




end

== matlab function Adap_ob_CIDA_3_ODR_CFC/Self Error Calculation 1/error_calculation ==
  data: v_di output; ref input; delta_x1 output; x_i input
function [v_di, delta_x1] = error_cal(ref, x_i)

%% Basic parameters

dimension = 3;
num_agent = 3;
serial_num = 1;

x_d = ref(1+dimension*0:dimension*num_agent);
v_d = ref(1+dimension*num_agent:2*dimension*num_agent);

x_di = x_d( (serial_num - 1)*dimension+1 : serial_num*dimension );
v_di = v_d( (serial_num - 1)*dimension+1 : serial_num*dimension );

delta_x1 = x_i - x_di;

end

== matlab function Adap_ob_CIDA_3_ODR_CFC/Controller and Plant 2/Controller/Auxiliary update ==
  data: u_nom input; xi_bar_dot output; u_sat input; g_i_hat input; xi_bar_i input
function xi_bar_dot = auxi_updata(u_nom, u_sat, g_i_hat, xi_bar_i)

eta_3 = diag([6,6,1]);

u_diff = u_nom - u_sat;

eta_4 = diag([0.5,0.5,0.2]);

% if norm(u_diff) == 0
%     eta_8 = diag([2,2,2]);
% else
%     eta_8 = diag([0.5,0.5,0.2]);
% end

xi_bar_dot = eta_3 * g_i_hat * u_diff - eta_4 * xi_bar_i;

end

== matlab function Adap_ob_CIDA_3_ODR_CFC/Controller and Plant 2/Controller/controller ==
  data: x_i input; v_di input; u_nom output; e_xi input; w_hat input; xi_bar_i input; g_i_hat output
function [u_nom, g_i_hat] = controller(x_i, v_di, e_xi, w_hat, xi_bar_i)

%% Reverse of the control gain matrix
Radius_esti=[0.13,0.13,0.13];

serial_num = 2;
dimension = 3; 

R_hat=Radius_esti(serial_num);

theta = x_i(dimension);

g_i_hat = [-sin(theta) -sin(pi/3 - theta) sin(pi/3 + theta);
        cos(theta) -cos(pi/3 - theta) -cos(pi/3+ theta);
        1/R_hat 1/R_hat 1/R_hat];

g_inverse = g_i_hat^(-1); 

%% Nominal control input
k_e = diag([1.6,1.6,1.6]);
k_xi = diag([8,8,2]);

u_nom = g_inverse * (- k_e * e_xi - k_xi * xi_bar_i - w_hat + v_di);

end

== matlab function Adap_ob_CIDA_3_ODR_CFC/Controller and Plant 1/Finite-time observer/Adaptive term/Update law ==
  data: x_tilde input; dot_E_hat output; E_hat_prev input
function dot_E_hat = adaptive_law(x_tilde, E_hat_prev)

eta_5 = diag([10,10,3]);
eta_6 = 1.1;
p = 9/11;
dot_E_hat = eta_5 * x_tilde - eta_6 * E_hat_prev;
% dot_E_hat = eta_5 * sign(x_tilde) .* abs(x_tilde).^(2*p-1);

end

== matlab function Adap_ob_CIDA_3_ODR_CFC/Controller and Plant 1/Estimation error ==
  data: E_i input; E_i_tilde output; E_i_hat input; E_tilde_norm output
function [E_i_tilde, E_tilde_norm] = esti_error(E_i, E_i_hat)

E_i_tilde = E_i - E_i_hat;
E_tilde_norm = norm(E_i_tilde);

end

== matlab function Adap_ob_CIDA_3_ODR_CFC/Controller and Plant 2/Estimation error ==
  data: E_i input; E_i_tilde output; E_i_hat input; E_tilde_norm output
function [E_i_tilde, E_tilde_norm] = esti_error(E_i, E_i_hat)

E_i_tilde = E_i - E_i_hat;
E_tilde_norm = norm(E_i_tilde);

end

== matlab function Adap_ob_CIDA_3_ODR_CFC/Controller and Plant 3/Estimation error ==
  data: E_i input; E_i_tilde output; E_i_hat input; E_tilde_norm output
function [E_i_tilde, E_tilde_norm] = esti_error(E_i, E_i_hat)

E_i_tilde = E_i - E_i_hat;
E_tilde_norm = norm(E_i_tilde);

end
